simulink model "LPV_model_NewBlock_R2024b"  (R2025b)
settings: Solver=VariableStepAuto  StartTime=0.0  StopTime=10.0  RelTol=1e-3
undefined symbols (not defined in the file or in its folder): G, M, Na, Nb, NBoccur, Nd, nDelta, nu, nx, nxMux, ny, str
settings Model: Creator=d.alazard  LastModifiedBy=andre

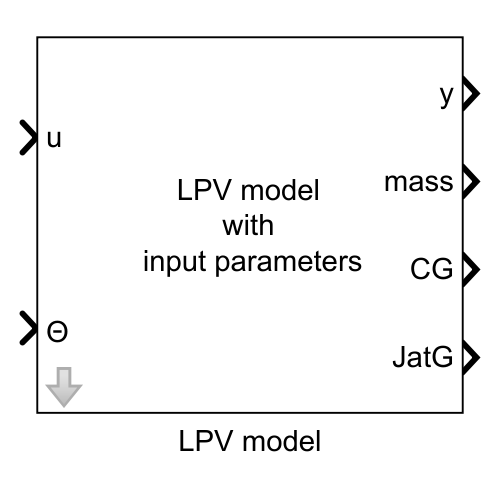
[thumbnail: Simulink's stored preview of the top-level diagram]
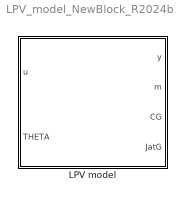
== system LPV_model_NewBlock_R2024b ==
  LPV model : Subsystem  mask(LPV model with input parameters){Gu=G, channelDCgain=1:6, channelInv=[7:9], RefreshG=Discrete, Tmodel=0.1, npt=0.01, TmodelSaved=0.1, nptSaved=0.01}
      mask prompts: Gu "Uncertain system (uss)"; channelDCgain "Channel corresponding to the transfer W_./C->Xddot_C (e.g. 1:6)"; channelInv "Channels to invert in the computation of the MCI"; RefreshG "Method"; Tmodel "Sampling period (second)"; npt "Normalized parameter variation threshold (>0 and  <1)"; TmodelSaved "Previous sampling period"; nptSaved "previous threshold"
      mask help:
      | This block implements an LPV model (uss generated with the SDTlib) with all the parameters defined by inputs.
      | It is assumed that:
      | * the LPV model Gu depends only on real parameters (ureal),
      | * the parameters on the second input of this block are ordered in the same order than the block description of Gu.
      |
      | Returns the outputs of the model, but also evolutions of the mass, center of gravity, and matrix of inertia. For this, it it necessary to specify which channels correspond to the transfer from input wrench (at a given point) to output accelerations. It is also possible to specify channels to invert. Typically, if the revolute joints of a robotic arm have torques as inputs and angular accelerations as outputs, these channels should be inverted.
      |
      | For faster simulation, it is recommended to update the model in discrete-time. In that case, it is also possible to update the model only when the variation of a normalized parameter (as provided by lfrdata) w.r.t. the previous update is greater that the "normalized parameter varaition thresold".
      |
      | Note that the "Continuous" and the "Inherit" update methods work only for MATLAB releases R2021a and later. They might require to activate an option: Model settings -> Simulation Target -> Advnced parameters -> Enable continuous-time MATLAB functions to write to initialized persistent variables
      |
      | Made by DYCSYT.
      mask init:
      | init_LPV_model
      mask TypeOptions RefreshG: Inherit | Discrete | Continuous
      mask Callback RefreshG: refreshG_callback
      mask DialogControl Container3 Prompt: Model Update
      mask Display:
      | disp('LPV model\nwith\n input parameters')
      | port_label('input', 1, 'u')
      | port_label('output', 1, 'y')
      | port_label('input',2,'\Theta','interpreter','tex')
      | port_label('output',2,'mass');
      | port_label('output',3,'CG');
      | port_label('output',4,'JatG');

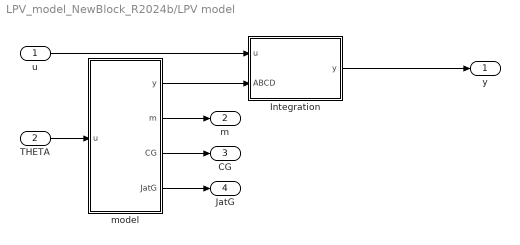
== system LPV_model_NewBlock_R2024b/LPV model ==
  u : Inport
  THETA : Inport  Port=2
  Integration : Subsystem
  model : MATLAB Function  TreatAsAtomicUnit=on  mask{ABCD=[M.a M.b;M.c M.d], nx=nx, nDelta=nDelta, NBoccur=NBoccur, str=str, Na=Na, Nb=Nb, Nd=Nd, npt=npt, yi=zeros(nx+ny,nx+nu), RefreshG=RefreshG, channelDCgain=channelDCgain, channelInv=channelInv}
      mask prompts: ABCD "SS matrics [M.a M.b;M.c M.d] (LFT model)"; nx "number of states nx (integer)"; nDelta "size of the Delta block"; NBoccur "Vecteur of occurrence numbers"; str "Uncertainty structure"; Na "Normalisation parameters Na (vector)"; Nb "Normalisation parameters Nb (vector)"; Nd "Normalisation parameters Nd (vector)"; npt "Normalized parameter variation threshold"; yi "initial value of the y"; RefreshG "Update Method (integer)"; channelDCgain "Channel corresponding to the transfer W_./C->Xddot_C (e.g. 1:6)"; channelInv "Channels to invert in the computation of the MCI"
  y : Outport
  m : Outport  Port=2
  CG : Outport  Port=3
  JatG : Outport  Port=4
  wires:
  THETA/1 -> model/1(u)
  model/2(m) -> m/1
  model/3(CG) -> CG/1
  model/4(JatG) -> JatG/1
  u/1 -> Integration/1(u)
  model/1(y) -> Integration/2(ABCD)
  Integration/1(y) -> y/1

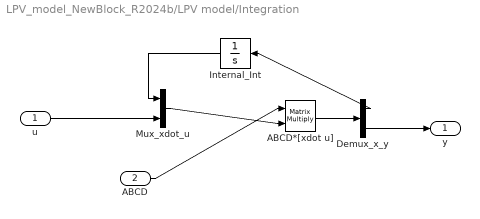
== system LPV_model_NewBlock_R2024b/LPV model/Integration ==
  u : Inport
  ABCD : Inport  Port=2
  ABCD*[xdot u] : Product  Multiplication=Matrix(*)
  Demux_x_y : Demux  Outputs=[nxMux ny]
  Internal_Int : Integrator
  Mux_xdot_u : Mux  Inputs=[nxMux nu]
  y : Outport
  wires:
  u/1 -> Mux_xdot_u/2
  Demux_x_y/2 -> y/1
  Mux_xdot_u/1 -> ABCD*[xdot u]/2
  ABCD*[xdot u]/1 -> Demux_x_y/1
  Internal_Int/1 -> Mux_xdot_u/1
  Demux_x_y/1 -> Internal_Int/1
  ABCD/1 -> ABCD*[xdot u]/1

== matlab function LPV_model_NewBlock_R2024b/LPV model/model ==
  settings: updateMethod=DISCRETE  sampleTime=Tmodel
  data: u input size=Nparam; y output size=[nx+ny,nx+nu]; ABCD parameter; nx parameter; nDelta parameter; NBoccur parameter; str parameter; Na parameter; Nb parameter; Nd parameter; npt parameter; yi parameter; RefreshG parameter; m output size=1; CG output size=3; JatG output size=[3,3]; channelDCgain parameter; channelInv parameter
function [y,m,CG,JatG]  = myfun(u,ABCD,nx,nDelta,NBoccur,str,Na,Nb,Nd,npt,yi,RefreshG,channelDCgain, channelInv)
y=yi;
% Normalization:
u=(Na+Nb.*u)./(1+Nd.*u);
persistent ABCDc p l
if RefreshG==2,
    if isempty(p);
        if length(NBoccur)~=length(u)
            disp('Wrong number of parameter inputs'),
        end
        l=size(ABCD,1);
        p=u;
        delta=u(1)*eye(NBoccur(1));
        for ii=2:length(u),
            delta=blkdiag(delta,u(ii)*eye(NBoccur(ii)));
        end
        ABCDc=[ABCD(:,1:nx) zeros(l,nDelta) ABCD(:,nx+nDelta+1:end)]+...
              ABCD(:,nx+1:nx+nDelta)*inv(eye(nDelta)-delta*ABCD(nx+1:nx+nDelta,nx+1:nx+nDelta))*...
              [delta*ABCD(nx+1:nx+nDelta,1:nx) eye(nDelta) delta*ABCD(nx+1:nx+nDelta,nx+nDelta+1:end)];
    else
        for ii=1:length(u);
            if abs(u(ii)-p(ii))>npt,
                ndii=NBoccur(ii);
                deltaii=(u(ii)-p(ii))*eye(ndii);
                ABCDc=[ABCDc(:,1:str(ii,1)-1) zeros(l,ndii) ABCDc(:,str(ii,2)+1:end)]+...
                ABCDc(:,str(ii,1):str(ii,2))*inv(eye(ndii)-deltaii*ABCDc(str(ii,1):str(ii,2),str(ii,1):str(ii,2)))*...
                [deltaii*ABCDc(str(ii,1):str(ii,2),1:str(ii,1)-1) eye(ndii) deltaii*ABCDc(str(ii,1):str(ii,2),str(ii,2)+1:end)];
                p(ii)=u(ii);
            end
        end
    end
else
    l=size(ABCD,1);
    delta=u(1)*eye(NBoccur(1));
    for ii=2:length(u),
        delta=blkdiag(delta,u(ii)*eye(NBoccur(ii)));
    end
    ABCDc=[ABCD(:,1:nx) zeros(l,nDelta) ABCD(:,nx+nDelta+1:end)]+...
          ABCD(:,nx+1:nx+nDelta)*inv(eye(nDelta)-delta*ABCD(nx+1:nx+nDelta,nx+1:nx+nDelta))*...
          [delta*ABCD(nx+1:nx+nDelta,1:nx) eye(nDelta) delta*ABCD(nx+1:nx+nDelta,nx+nDelta+1:end)];    
end
y(1:end,1:end) = ABCDc([1:nx nx+nDelta+1:end],[1:nx nx+nDelta+1:end]);
% % To compute MCI it is assumed that the first 6 outputs are the
% % accelerations of the main body at the point C (defined in the SDTlib
% % model) and the fisrt 6 inputs is the wrench appled at the point C.
% % Massm1=y(nx+1:end,nx+1:end)-y(nx+1:end,1:nx)*inv(y(1:nx,1:nx))*y(1:nx,nx+1:end);

% % Modification: the user can select the channels to compute the dcgain
% and also which channels should be inverted (here the transfer between the
% input torques of the robotic arm and the output angular accelerations)
if channelInv~=0,
          ind = channelInv;
          A = y(1:nx,1:nx); B = y(1:nx,nx+1:end); C = y(nx+1:end,1:nx); D = y(nx+1:end,nx+1:end);
          in1=setdiff(1:size(B,2),ind);
          in2=ind;
          out1=setdiff(1:size(C,1),ind);
          out2=ind;
          B1=B(:,in1);B2=B(:,in2);
          C1=C(out1,:);C2=C(out2,:);
          D11=D(out1,in1);D12=D(out1,in2);D21=D(out2,in1);D22=D(out2,in2);
          if cond(D22)==Inf, 
              warning('The channels to be inverted in the LPV plant are not invertible. MCI properties might be incorrect.')
              y_inv = y;
          else
              D22i=inv(D22);
              y_inv = [A-B2*D22i*C2, [B1-B2*D22i*D21 B2*D22i]; [C1-D12*D22i*C2;-D22i*C2], [D11-D12*D22i*D21 D12*D22i;-D22i*D21 D22i]];
          end
else
          y_inv = y;
end
Massm1=y_inv(nx+(channelDCgain),nx+(channelDCgain))-y_inv(nx+(channelDCgain),1:nx)*inv(y_inv(1:nx,1:nx))*y_inv(1:nx,nx+(channelDCgain));
Mass=inv(Massm1);
m=Mass(1,1);
if abs(Mass(1,1) - Mass(2,2)) > 1e-5 || abs(Mass(1,1) - Mass(3,3)) > 1e-5 || abs(Mass(2,2) - Mass(3,3)) > 1e-5 % some tolerance of 1e-5 when checking equality
    warning('The mass matrix has different values on its diagonal (whereas all 3 terms should be equal to the mass). The MCI properties might be incorrect. This might come from an error in field "Channels to invert"')
end
CG=[Mass(2,6);-Mass(1,6);Mass(1,5)]/m;
JatG=Mass(4:6,4:6)+m*antisym(CG)^2;
end
